simulink model "pos_control2_test"  (R2016b)
settings: Solver=ode3  StartTime=0.0  StopTime=30  FixedStep=0.0025  RelTol=1e-3
model workspace: external: MATLAB File /home/hywel/Simulink/2017_10_drone/para_pos.m (data not in the file)
undefined symbols (not defined in the file or in its folder): bool_pos, control_mode, def, par, par_input, par_pos, position_setpoint, v_control_mode
(part 2 of 2)

== matlab function pos_control2_test/position_control/control_position ==
  data: vel_sp_prev_x input; vel_sp_prev_y input; vel_sp_prev_z input; pos_sp_prev_x input; pos_sp_prev_y input; pos_sp_prev_z input; pos input; vel input; curr_pos_sp input; att_euler input; vehicle_land_detected input; takeoff_vel_limit input; att_sp_yaw_body input; vel_max_xy input; vel_sp output; pos_sp output; att_sp output; att_sp_3 output; local_pos_sp_acc output; judge_auto_enable output; thrust_int_prev input; State_prev input; input_prev input; v_err_d input; thrust_int output; def parameter; bool_pos parameter; par_pos parameter; control_mode parameter; par_input parameter; position_setpoint parameter; State output; input output; thrust_sp output; saturation_xy output; saturation_z output; vel_err output; testbool output; thrust_body_z output; R_z output; R_set_output output; body_z output; dt input
function [vel_sp,pos_sp,att_sp,att_sp_3,local_pos_sp_acc,judge_auto_enable,thrust_int,State,input,thrust_sp,saturation_xy,saturation_z,vel_err,testbool,thrust_body_z,R_z,R_set_output,body_z] = control_position(vel_sp_prev_x,vel_sp_prev_y,vel_sp_prev_z, pos_sp_prev_x,pos_sp_prev_y,pos_sp_prev_z, pos, vel, curr_pos_sp, att_euler, vehicle_land_detected, takeoff_vel_limit, att_sp_yaw_body,vel_max_xy, thrust_int_prev,State_prev,input_prev, v_err_d,def, bool_pos, par_pos, control_mode, par_input, position_setpoint,dt)
% run position & altitude controllers, if enabled (otherwise use already computed velocity setpoints) */
% prev_pos_sp(x,y,z,type,yaw_valid,yawspeed_valid,yaw,yawspeed,cruising_speed,cruising_valid,acceleration_valid,ax,ay,az)
%prev_pos_sp(valid,type,x,y,z,vx,vy,vz,ax,ay,az,yaw,yawspeed,cruising_speed,position_valid,velocity_valid,acceleration_valid,yaw_valid,yawspeed_valid,cruising_valid)

% vehicle_land_detected(bool_landed,bool_freeall,bool_ground_contact,bool_maybe_landed,alt_max)
%[0]
%att_sp(roll_body,pitch_body,yaw_body,q1_d,q2_d,q3_d,q4_d,thrust,q_d_valid)
%_takeoff_vel_limit = 0.5
body_z = zeros(3,1);
input = zeros(3,1);
R_set_output = zeros(9,1);
vel_err = zeros(3,1);
thrust_sp = zeros(3,1);
R_z = zeros(3,1);
thrust_body_z = 0;
%bool 
saturation_xy = 0;
%bool 
saturation_z = 0;
testbool = bool_pos.reset_int_xy;

vel_sp_prev = [vel_sp_prev_x,vel_sp_prev_y,vel_sp_prev_z]';
pos_sp_prev = [pos_sp_prev_x,pos_sp_prev_y,pos_sp_prev_z];
pos_sp = pos_sp_prev;
vel_sp = vel_sp_prev;
State = State_prev;

thrust_int = thrust_int_prev;
att_sp = zeros(9,1);
att_sp_3 = zeros(3,1);
att_sp(3) = att_sp_yaw_body;
R = euler_to_dcm(att_euler);
R_setpoint = zeros(3,3);
local_pos_sp_acc = zeros(3,1);
judge_auto_enable = 1;

if (bool_pos.run_pos_control)
    % If for any reason, we get a NaN position setpoint, we better just stay where we are.
    if (isreal(pos_sp(1)) && isreal(pos_sp(2)))
        vel_sp(1) = (pos_sp(1) - pos(1)) * par_pos.pos_p(1);
        vel_sp(2) = (pos_sp(2) - pos(2)) * par_pos.pos_p(2);
    else
        vel_sp(1) = 0.0;
        vel_sp(2) = 0.0;
        %warn_rate_limited("Caught invalid pos_sp in x and y");
    end
end

% in auto the setpoint is already limited by the navigator */

if (~control_mode.flag_control_auto_enabled)
    %limit_altitude();
    
    if (vehicle_land_detected(5) < 0.0)
        judge_auto_enable = 0;
    % there is no altitude limitation present
    %return;
    end

    %float 
    altitude_above_home = -(pos(3) - par_input.home_pos(3));

    if (bool_pos.run_alt_control && (altitude_above_home > vehicle_land_detected(5)))
        % we are above maximum altitude
        pos_sp(3) = -vehicle_land_detected(5) +  par_input.home_pos(3);

    elseif (~bool_pos.run_alt_control && vel_sp(3) <= 0.0)
        % we want to fly upwards: check if vehicle does not exceed altitude

        % time to reach zero velocity
        %float 
        delta_t = -vel(3) / par_pos.acceleration_z_max_down;

        % predict next position based on current position, velocity, max acceleration downwards and time to reach zero velocity
        %float 
        pos_z_next = pos(3) + vel(3) * delta_t + 0.5 * par_pos.acceleration_z_max_down * delta_t *delta_t;

        if (-(pos_z_next - par_input.home_pos(3)) > vehicle_land_detected(5))
            % prevent the vehicle from exceeding maximum altitude by switching back to altitude control with maximum altitude as setpoint
            pos_sp(3) = -vehicle_land_detected(5) + par_input.home_pos(3);
            % test 
            %bool_pos.run_alt_control = 1;
        end
    end
end

if (bool_pos.run_alt_control)
    if (isreal(pos_sp(3)))
        vel_sp(3) = (pos_sp(3) - pos(3)) * par_pos.pos_p(3);

    else
        vel_sp(3) = 0.0;
        %warn_rate_limited("Caught invalid pos_sp in z");
    end
end


if (~control_mode.flag_control_position_enabled)
    %bool_pos.reset_pos_sp = 1;
end

if (~control_mode.flag_control_altitude_enabled)
    %bool_pos.reset_alt_sp = 1;
end

if (~control_mode.flag_control_velocity_enabled)
    %vel_sp_prev(1) = vel(1);
    %vel_sp_prev(2) = vel(2);
    vel_sp(1) = 0.0;
    vel_sp(2) = 0.0;
end

if (~control_mode.flag_control_climb_rate_enabled)
    vel_sp(3) = 0.0;
end

% limit vertical upwards speed in auto takeoff and close to ground */
%float 
altitude_above_home = -pos(3) + par_input.home_pos(3);

if (curr_pos_sp(2) == position_setpoint.SETPOINT_TYPE_TAKEOFF && ~control_mode.flag_control_manual_enabled)
    %float 
    vel_limit = gradual(altitude_above_home, par_pos.slow_land_alt2, par_pos.slow_land_alt1, par_pos.tko_speed, par_pos.vel_max_up);
    vel_sp(3) = max(vel_sp(3), -vel_limit);
end

% limit vertical downwards speed (positive z) close to ground
% for now we use the altitude above home and assume that we want to land at same height as we took off */
%float 
vel_limit = gradual(altitude_above_home, par_pos.slow_land_alt2, par_pos.slow_land_alt1, par_pos.land_speed, par_pos.vel_max_down);

vel_sp(3) = min(vel_sp(3), vel_limit);

% apply slewrate (aka acceleration limit) for smooth flying */

if (~control_mode.flag_control_auto_enabled)
    %todo
    %vel_sp_slewrate(dt);
    %matrix::Vector2f 
    vel_sp_xy = [vel_sp(1), vel_sp(2)]';
	%matrix::Vector2f 
    vel_sp_prev_xy = [vel_sp_prev(1), vel_sp_prev(2)]';
	%matrix::Vector2f 
    vel_xy = [vel(1), vel(2)]';
	%matrix::Vector2f 
    acc_xy = (vel_sp_xy - vel_sp_prev_xy)/ dt;

	% limit total horizontal acceleration */
    if (normest(acc_xy) > par_pos.acceleration_state_dependent_xy)
		vel_sp_xy = par_pos.acceleration_state_dependent_xy * acc_xy/normest(acc_xy) * dt + vel_sp_prev_xy;
		vel_sp(1) = vel_sp_xy(1);
		vel_sp(2) = vel_sp_xy(2);
    end

	% limit vertical acceleration */
	%float 
    acc_z = (vel_sp(3) - vel_sp_prev(3)) / dt;
	%float 
    %max_acc_z;

    if (control_mode.flag_control_manual_enabled)
        if acc_z < 0.0
            max_acc_z = -par_pos.acceleration_state_dependent_z;
        else
            max_acc_z = par_pos.acceleration_state_dependent_z;
        end
    else
        if acc_z < 0.0
            max_acc_z = -par_pos.acceleration_z_max_up;
        else
            max_acc_z = par_pos.acceleration_z_max_up;
        end
    end
    
    if (abs(acc_z) > abs(max_acc_z))
		vel_sp(3) = max_acc_z * dt + vel_sp_prev(3);
    end
end

%vel_sp_prev = vel_sp;

% special velocity setpoint limitation for smooth takeoff (after slewrate!) */
if (bool_pos.in_smooth_takeoff)
    if (takeoff_vel_limit < -vel_sp(3))
        %bool_pos.in_smooth_takeoff = 1;
    else
        %bool_pos.in_smooth_takeoff = 0;
    end
    % ramp vertical velocity limit up to takeoff speed */
    takeoff_vel_limit = takeoff_vel_limit -vel_sp(3) * dt / par_pos.takeoff_ramp_time;
    % limit vertical velocity to the current ramp value */
    vel_sp(3) = max(vel_sp(3), -takeoff_vel_limit);
end

% make sure velocity setpoint is constrained in all directions (xyz) */
%float 
vel_norm_xy = sqrt(vel_sp(1) * vel_sp(1) + vel_sp(2) * vel_sp(2));

if (vel_norm_xy > vel_max_xy) 
    vel_sp(1) = vel_sp(1) * vel_max_xy / vel_norm_xy;
    vel_sp(2) = vel_sp(2) * vel_max_xy / vel_norm_xy;
end

vel_sp(3) = constrain(vel_sp(3), -par_pos.vel_max_up, par_pos.vel_max_down);


if (control_mode.flag_control_climb_rate_enabled || control_mode.flag_control_velocity_enabled || control_mode.flag_control_acceleration_enabled)
    	% reset integrals if needed */
    if (control_mode.flag_control_climb_rate_enabled)
        if (bool_pos.reset_int_z)
            %bool_pos.reset_int_z = 0;
            thrust_int(3) = 0.0;
        end
    else
        %bool_pos.reset_int_z = 1;
    end

    if (control_mode.flag_control_velocity_enabled)
        if (bool_pos.reset_int_xy)
            %bool_pos.reset_int_xy = 0;
            thrust_int(1) = 0.0;
            thrust_int(2) = 0.0;
        end
    else
        %bool_pos.reset_int_xy = 1;
    end

    % if any of the velocity setpoint is bogus, it's probably safest to command no velocity at all. */
    for i = 1:3
        if (~isreal(vel_sp(i)))
            vel_sp(i) = 0.0;
        end
    end

    % velocity error */
    vel_err = vel_sp - vel;

    % thrust vector in NED frame */
    thrust_sp = zeros(3,1);
    
    %if (_control_mode.flag_control_acceleration_enabled && _pos_sp_triplet.current.acceleration_valid) {
    %thrust_sp = math::Vector<3>(_pos_sp_triplet.current.a_x, _pos_sp_triplet.current.a_y, _pos_sp_triplet.current.a_z);
    if (control_mode.flag_control_acceleration_enabled && curr_pos_sp(17))
        thrust_sp = [curr_pos_sp(9), curr_pos_sp(10), curr_pos_sp(11)]';
    else
        %todo
        %float 
        %float 
        input = -[vel(1),vel(2),vel(3)]';
        input2 = (input-input_prev)/dt;
        
        b = 2 * def.M_PI_F * 5 * dt;
        %float 
        a = b / (1 + b);
        %set
        State = (a * input2 + (1 - a)*State_prev);
        
        %vel_err_d = State;
        vel_err_d = v_err_d;
        thrust_sp = vel_err.*(par_pos.vel_p) + vel_err_d.*(par_pos.vel_d) + thrust_int - [0, 0, par_pos.thr_hover]';
    end

    if (~control_mode.flag_control_velocity_enabled && ~control_mode.flag_control_acceleration_enabled)
        thrust_sp(1) = 0.0;
        thrust_sp(2) = 0.0;
    end
    
    %bool
    in_auto_takeoff =  (curr_pos_sp(2) == position_setpoint.SETPOINT_TYPE_TAKEOFF) || control_mode.flag_control_offboard_enabled;
    %bool
    %todo has no maunal input
    has_manual_control_present = control_mode.flag_control_manual_enabled; % && manual.timestamp > 0;
	% Manual takeoff is triggered if the throttle stick is above 65%.
	manual_wants_takeoff = has_manual_control_present; % && manual.z > 0.65;
    
    if (~in_auto_takeoff && ~manual_wants_takeoff)
        if (vehicle_land_detected(3))
            % if still or already on ground command zero xy thrust_sp in body
            % frame to consider uneven ground */

            % thrust setpoint in body frame*/
            %math::Vector<3> 
            thrust_sp_body = R' * thrust_sp;

            % we dont want to make any correction in body x and y*/
            thrust_sp_body(1) = 0.0;
            thrust_sp_body(2) = 0.0;

            % make sure z component of thrust_sp_body is larger than 0 (positive thrust is downward) */
            if thrust_sp(3) > 0.0
                thrust_sp_body(3) = thrust_sp(3);
            else
                thrust_sp_body(3) = 0;
            end

            % convert back to local frame (NED) */
            thrust_sp = R * thrust_sp_body;
        end

        if (vehicle_land_detected(4))
            % we set thrust to zero
            % this will help to decide if we are actually landed or not
            
            thrust_sp = zeros(3,1);
        end
    end

    if (~control_mode.flag_control_climb_rate_enabled && ~control_mode.flag_control_acceleration_enabled)
        thrust_sp(3) = 0.0;
    end

    % limit thrust vector and check for saturation */
    %bool 
    saturation_xy = 0;
    %bool 
    saturation_z = 0;

    % limit min lift */
    %float 
    thr_min = par_pos.thr_min;

    if (~control_mode.flag_control_velocity_enabled && thr_min < 0.0)
        % don't allow downside thrust direction in manual attitude mode */
        thr_min = 0.0;
    end

    %float 
    tilt_max = par_pos.tilt_max_air;
    %float 
    thr_max = par_pos.thr_max;

    % We can only run the control if we're already in-air, have a takeoff setpoint,
    % or if we're in offboard control.
    % Otherwise, we should just bail out
    if (vehicle_land_detected(1) && ~in_auto_takeoff && ~manual_wants_takeoff)
        % Keep throttle low while still on ground.
        thr_max = 0.0;

    elseif (~control_mode.flag_control_manual_enabled && curr_pos_sp(2) == position_setpoint.SETPOINT_TYPE_LAND)
        % adjust limits for landing mode */
        % limit max tilt and min lift when landing */
        tilt_max = par_pos.tilt_max_land;
    end

    % limit min lift */
    if (-thrust_sp(3) < thr_min)
        thrust_sp(3) = -thr_min;
        % Don't freeze altitude integral if it wants to throttle up */
        if vel_err(3) > 0.0
            saturation_z = 1;
        end
    end

    if (control_mode.flag_control_velocity_enabled || control_mode.flag_control_acceleration_enabled)

        % limit max tilt */
        if (thr_min >= 0.0 && tilt_max < def.M_PI_F / 2 - 0.05)
            % absolute horizontal thrust */
            %float 
            thrust_sp_xy_len = normest([thrust_sp(1), thrust_sp(2)]);

            if (thrust_sp_xy_len > 0.01)
                % max horizontal thrust for given vertical thrust*/
                %float 
                thrust_xy_max = -thrust_sp(3) * tan(tilt_max);

                if (thrust_sp_xy_len > thrust_xy_max)
                    %float 
                    k = thrust_xy_max / thrust_sp_xy_len;
                    thrust_sp(1) = thrust_sp(1)*k;
                    thrust_sp(2) = thrust_sp(2)*k;
                    % Don't freeze x,y integrals if they both want to throttle down */
                    if (vel_err(1) * vel_sp(1) < 0.0) && (vel_err(2) * vel_sp(2) < 0.0)
                    else
                        saturation_xy = 1;
                    end
                end
            end
        end
    end


    if (control_mode.flag_control_climb_rate_enabled && ~control_mode.flag_control_velocity_enabled)
        % thrust compensation when vertical velocity but not horizontal velocity is controlled */
        %float 
        %att_comp;

        %const float 
        tilt_cos_max = 0.7;

        if (R(3, 3) > tilt_cos_max)
            att_comp = 1.0 / R(3, 3);

        elseif (R(3, 3) > 0.0)
            att_comp = ((1.0 / tilt_cos_max - 1.0) / tilt_cos_max) * R(3, 3) + 1.0;
            saturation_z = 1;

        else
            att_comp = 1.0;
            saturation_z = 1;
        end

        thrust_sp(3) =thrust_sp(3)* att_comp;
    end
    

    % Calculate desired total thrust amount in body z direction. */
    % To compensate for excess thrust during attitude tracking errors we
    % project the desired thrust force vector F onto the real vehicle's thrust axis in NED:
    % body thrust axis [0,0,-1]' rotated by R is: R*[0,0,-1]' = -R_z */
    %matrix::Vector3f 
    R_z=[R(1, 3), R(2, 3), R(3, 3)]';
    %matrix::Vector3f 
    F = thrust_sp;
    %float 
    thrust_body_z = dot(F, -R_z); % recalculate because it might have changed */

    % limit max thrust */
    if (abs(thrust_body_z) > thr_max)
        if (thrust_sp(3) < 0.0)
            if (-thrust_sp(3) > thr_max)
                % thrust Z component is too large, limit it */
                thrust_sp(1) = 0.0;
                thrust_sp(2) = 0.0;
                thrust_sp(3) = -thr_max;
                saturation_xy = 1;
                % Don't freeze altitude integral if it wants to throttle down */
                if vel_err(3) < 0.0
                    saturation_z = 1;
                end
            else
                % preserve thrust Z component and lower XY, keeping altitude is more important than position */
                %float 
                thrust_xy_max = sqrt(thr_max * thr_max - thrust_sp(3) * thrust_sp(3));
                %float 
                thrust_xy_abs = normest([thrust_sp(1), thrust_sp(2)]);
                %float 
                k = thrust_xy_max / thrust_xy_abs;
                thrust_sp(1) = thrust_sp(1)*k;
                thrust_sp(2) = thrust_sp(2)*k;
                % Don't freeze x,y integrals if they both want to throttle down */
                if (vel_err(1) * vel_sp(1) < 0.0) && (vel_err(2) * vel_sp(2) < 0.0)
                else
                    saturation_xy = 1;
                end
            end
        else
            % Z component is positive, going down (Z is positive down in NED), simply limit thrust vector */
            %float 
            k = thr_max / abs(thrust_body_z);
            thrust_sp = thrust_sp*k;
            saturation_xy = 1;
            saturation_z = 1;
        end
        thrust_body_z = thr_max;
    end

    % if any of the thrust setpoint is bogus, send out a warning */
    %if (~PX4_ISFINITE(thrust_sp(0)) || ~PX4_ISFINITE(thrust_sp(1)) || ~PX4_ISFINITE(thrust_sp(2)))
        %warn_rate_limited("Thrust setpoint not finite");
    % end

    %_att_sp.thrust
    att_sp(8) = max(thrust_body_z, thr_min);

    % update integrals */
    if (control_mode.flag_control_velocity_enabled && ~saturation_xy)
        thrust_int(1) = thrust_int(1) + vel_err(1) * par_pos.vel_i(1) * dt;
        thrust_int(2) = thrust_int(2) + vel_err(2) * par_pos.vel_i(2) * dt;
    end

    if (control_mode.flag_control_climb_rate_enabled && ~saturation_z)
        thrust_int(3) = thrust_int(3) + vel_err(3) * par_pos.vel_i(3) * dt;
    end

    % calculate attitude setpoint from thrust vector */
    if (control_mode.flag_control_velocity_enabled || control_mode.flag_control_acceleration_enabled)
        % desired body_z axis = -normalize(thrust_vector) */
        %math::Vector<3> 
        body_x = zeros(3,1);
        %math::Vector<3> 
        body_y = zeros(3,1);
        %math::Vector<3> 
        body_z = zeros(3,1);

        if (normest(thrust_sp) > def.SIGMA_NORM)
            body_z = -thrust_sp/normest(thrust_sp);

        else
            % no thrust, set Z axis to safe value */
            body_z = zeros(3,1);
            body_z(3) = 1.0;
        end

        % vector of desired yaw direction in XY plane, rotated by PI/2 */
        %math::Vector<3> 
        y_C = [-sin(att_sp(3)), cos(att_sp(3)), 0.0]';

        if (abs(body_z(3)) > def.SIGMA_SINGLE_OP)
            % desired body_x axis, orthogonal to body_z */
            body_x = cross(y_C, body_z);

            % keep nose to front while inverted upside down */
            if (body_z(3) < 0.0)
                body_x = -body_x;
            end

            body_x = body_x/normest(body_x);

        else
            % desired thrust is in XY plane, set X downside to construct correct matrix,
            % but yaw component will not be used actually */
            body_x = zeros(3,1);
            body_x(3) = 1.0;
        end

        % desired body_y axis */
        body_y = cross(body_z, body_x);

        % fill rotation matrix */
        for i = 1:3
            R_setpoint(i, 1) = body_x(i);
            R_setpoint(i, 2) = body_y(i);
            R_setpoint(i, 3) = body_z(i);
        end
        
        R_set_output(1) = R_setpoint(1, 1);
        R_set_output(2) = R_setpoint(1, 2);
        R_set_output(3) = R_setpoint(1, 3);
        R_set_output(4) = R_setpoint(2, 1);
        R_set_output(5) = R_setpoint(2, 2);
        R_set_output(6) = R_setpoint(2, 3);
        R_set_output(7) = R_setpoint(3, 1);
        R_set_output(8) = R_setpoint(3, 2);
        R_set_output(9) = R_setpoint(3, 3);
        % copy quaternion setpoint to attitude setpoint topic */
        %matrix::Quatf 
        q_sp = dcm_to_q(R_setpoint);
        att_sp(4) = q_sp(1);
        att_sp(5) = q_sp(2);
        att_sp(6) = q_sp(3);
        att_sp(7) = q_sp(4);
        att_sp(9) = 1;

        % calculate euler angles, for logging only, must not be used for control */
        %matrix::Eulerf 
        euler = dcm_to_euler(R_setpoint);
        att_sp(1) = euler(1);
        att_sp(2) = euler(2);
        % yaw already used to construct rot matrix, but actual rotation matrix can have different yaw near singularity */

    elseif (~control_mode.flag_control_manual_enabled)
        % autonomous altitude control without position control (failsafe landing),
        % force level attitude, don't change yaw */
        R_setpoint = euler_to_dcm([0.0, 0.0, att_sp(3)]);

        % copy quaternion setpoint to attitude setpoint topic */
        %matrix::Quatf 
        q_sp = q_to_dcm(R_setpoint);
        att_sp(4) = q_sp(1);
        att_sp(5) = q_sp(2);
        att_sp(6) = q_sp(3);
        att_sp(7) = q_sp(4);
        
        att_sp(9) = 1;

        att_sp(1) = 0.0;
        att_sp(2) = 0.0;
    end

    % save thrust setpoint for logging */
    
    local_pos_sp_acc(1) = thrust_sp(1) * def.CONSTANTS_ONE_G;
    local_pos_sp_acc(2)= thrust_sp(2) * def.CONSTANTS_ONE_G;
    local_pos_sp_acc(3) = thrust_sp(3) * def.CONSTANTS_ONE_G;

    %_att_sp.timestamp = hrt_absolute_time();

else
    %bool_pos.reset_int_z = 1;
end

att_sp_3(1) = att_sp(1);
att_sp_3(2) = att_sp(2);
att_sp_3(3) = att_sp(3);
